simulink model "ImpulseSDOF_1Pedestrian_sim"  (R2022a)
settings: Solver=ode4  StartTime=t_inicial  StopTime=t_final  FixedStep=t_step  RelTol=1e-3
values from neighbouring files (symbols this model uses):
  A = [0 1; -Kbridge/Mbridge -Cbridge/Mbridge]    [ImpulseSDOF_1Pedestrian.m]
  ai = 1    [ImpulseSDOF_1Pedestrian.m]    (also in Impulse_vdpWalkerB2017.m; TeastingvdPWalker_B2017.m; TestingvdPWalker_B2017.m)
  B = [0; -ped_mass/Mbridge]    [ImpulseSDOF_1Pedestrian.m]
  C = [1 0; 0 1; -Kbridge/Mbridge -Cbridge/Mbridge]    [ImpulseSDOF_1Pedestrian.m]
  D = [0;0;-ped_mass/Mbridge]    [ImpulseSDOF_1Pedestrian.m]
  lambdai = 0.23    [ImpulseSDOF_1Pedestrian.m]    (also in Impulse_vdpWalkerB2017.m; TeastingvdPWalker_B2017.m; TestingvdPWalker_B2017.m)
  ped_mass = 70    [ImpulseSDOF_1Pedestrian.m]
  wi = 0.75    [ImpulseSDOF_1Pedestrian.m]    (also in Impulse_vdpWalkerB2017.m; TeastingvdPWalker_B2017.m = 0.73; TestingvdPWalker_B2017.m)
libraries: cstblocks x1
settings Model: Creator=Javiera  LastModifiedBy=LEGION
settings SolverCC: AlgebraicLoopSolver=TrustRegion
settings DebuggingCC: UnconnectedInputMsg=warning  UnconnectedOutputMsg=warning  UnconnectedLineMsg=warning  SFMachineParentedDataDiag=warning

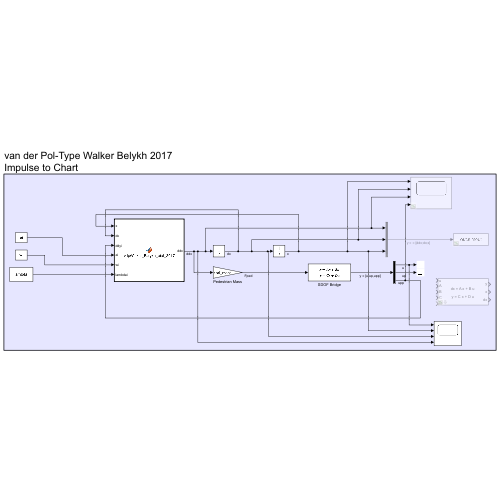
[thumbnail: Simulink's stored preview of the top-level diagram]
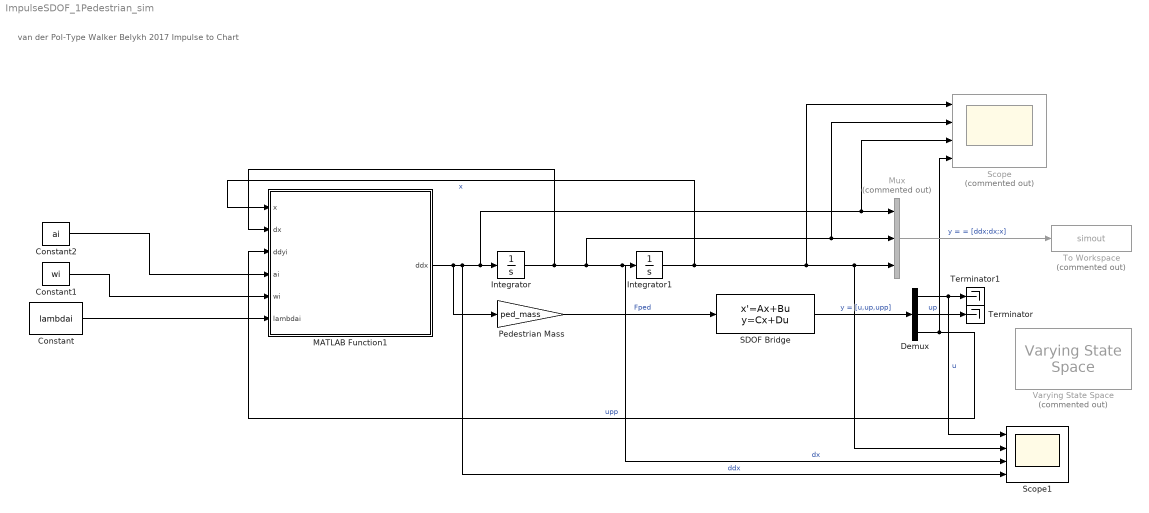
== system ImpulseSDOF_1Pedestrian_sim ==
  note: van der Pol-Type Walker Belykh 2017
      | Impulse to Chart
  Constant : Constant  Value=lambdai
  Constant1 : Constant  Value=wi
  Constant2 : Constant  Value=ai
  Demux : Demux  Outputs=3
  Integrator : Integrator
  Integrator1 : Integrator
  MATLAB Function1 : MATLAB Function  TreatAsAtomicUnit=on
  Mux : Mux  Commented=on  Inputs=3
  Pedestrian Mass : Gain  Gain=ped_mass
  SDOF Bridge : StateSpace  A=A  B=B  C=C  D=D  InitialCondition=0.05
  Scope : Scope  Commented=on  NumInputPorts=4
  Scope1 : Scope  NumInputPorts=4
  Terminator : Terminator
  Terminator1 : Terminator
  To Workspace : ToWorkspace  Commented=on  VariableName=simout  SaveFormat=Timeseries  SampleTime=-1
  Varying State Space : cstblocks/Linear Parameter Varying/Varying State Space  Commented=on  x0=0  xNames=''  OutputX=on  OutputDX=on
  wires:
  MATLAB Function1/1(ddx) -> Scope1/4, Scope/3, Mux/1, Integrator/1, Pedestrian Mass/1  "ddx"
  Integrator/1 -> MATLAB Function1/2(dx), Scope1/3, Integrator1/1, Scope/2, Mux/2  "dx"
  Integrator1/1 -> Scope1/2, Mux/3, Scope/1, MATLAB Function1/1(x)  "x"
  Demux/3 -> Scope/4, MATLAB Function1/3(ddyi)  "upp"
  SDOF Bridge/1 -> Demux/1  "y = [u,up,upp]"
  Demux/2 -> Terminator/1  "up"
  Demux/1 -> Scope1/1, Terminator1/1  "u"
  Mux/1 -> To Workspace/1  "y = = [ddx;dx;x]"
  Constant2/1 -> MATLAB Function1/4(ai)
  Constant1/1 -> MATLAB Function1/5(wi)
  Constant/1 -> MATLAB Function1/6(lambdai)
  Pedestrian Mass/1 -> SDOF Bridge/1  "Fped"

== matlab function ImpulseSDOF_1Pedestrian_sim/MATLAB Function1 ==
  data: x input; ddx output; dx input; ddyi input; ai input; wi input; lambdai input
function ddx = vdpWalker_Belykh_etal_2017(x,dx,ddyi,ai,wi,lambdai)
% Alexis Contreras R. 

% Foot force models of crowd dynamics on a wobbly bridge
% Igor V. Belykh, Russel Jeter and Vladimir N. Belykh (2017)

% Modelo de peatón de oscilador auto-sostenible donde los pasos se ajustan
% al movimiento del puente. El balance humano se modela como péndulo invertido.
% de la forma de oscilador van der Pol (vdP)

%%%%%%%%%%%%%%%%%%%%%%%%%%%%%%%%%%%%%%%%%%%%%%%%%%%%%%%%%%%%%%%%%%%%%%%%%%%
% Inputs:
% x         -> Desplazamiento del centro de masa (CoM) del peatón
% dx        -> Velocidad del centro de masa del peatón 
% ddyi      -> Aceleración absoluta del puente (o relativa al suelo/punto fijo externo)
% lambdai   -> Parámetro de amortiguamiento
% ai        -> Parámetro de control del mecanismo de auto-excitación del caminar humano
% wi        -> wi = sqrt(g/L), del modelo pendulo invertido (L >> x)

% Outputs:
% ddx       -> Aceleración del peatón
%%%%%%%%%%%%%%%%%%%%%%%%%%%%%%%%%%%%%%%%%%%%%%%%%%%%%%%%%%%%%%%%%%%%%%%%%%%
% fxdx = lambdai*(dx^2-vi^2*x^2+vi^2*ai^2)*dxi-w0^2*xi; (Eq.4)

fxdx = lambdai*(dx^2 + x^2 + ai^2)*x + wi^2*x;                                  % (Eq.5)
ddx = -ddyi - fxdx;                                                         % (Eq.1)
